simulink model "Robot2"  (R2019b)
settings: Solver=ode4  StartTime=0.0  StopTime=Tsim  FixedStep=Ts  RelTol=1e-3
values from neighbouring files (symbols this model uses):
  alfa = 20    [MAIN.m]
  delta = 0.1    [MAIN.m]
  gain = 1.0    (= 1)    [MAIN.m]
  Gname = ['G' num2str(grados) 'Rn']    [MAIN.m]
  IMname = ['InvMass' num2str(grados) 'Rn' ]    [MAIN.m]
  K = 0.1    [MAIN.m]
  lambda = 20    [MAIN.m]
  limD = -[60 40]'    [MAIN.m]
  limU = [60 40]'    [MAIN.m]
  Mname = ['Mass' num2str(grados) 'Rn' ]    [MAIN.m]
  P = 1    [MAIN.m]
  q0 = [0 0]'    [MAIN.m]
  q01 = q0+(Offset*pi/180)    [MAIN.m]
  qd0 = [0 0]'    [MAIN.m]
  Tg = 1e-3    (= 0.001)    [MAIN.m]
  Vname = ['V' num2str(grados) 'Rn' ]    [MAIN.m]
undefined symbols (not defined in the file or in its folder): smiData, X, Y, Z
libraries: sm_lib x16, nesl_utility x7
settings Model: Creator=AP34340  LastModifiedBy=AP34340
settings DataIOCC: SaveOutput=off  SignalLogging=off  DSMLogging=off  SaveTime=off  ReturnWorkspaceOutputs=off
settings OptimizationCC: LifeSpan=inf
settings DebuggingCC: SFExecutionAtInitializationDiag=none  ArithmeticOperatorsInVariantConditions=warning
settings HardwareCC: ProdBitPerSizeT=32  ProdBitPerPtrDiffT=32  ProdWordSize=32  ProdHWDeviceType=Specified
settings ModelReferenceCC: EnableParallelModelReferenceBuilds=on  ParallelModelReferenceMATLABWorkerInit=Load Top Model
settings SFSimCC: CustomCodeUndefinedFunction=UseInterfaceOnly
settings CodeAppCC: StateflowObjectComments=on
settings SimscapeCC: SimscapeNormalizeSystem=off

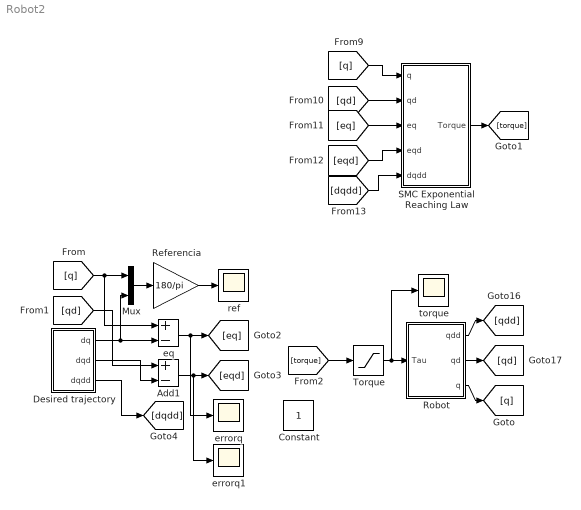
== system Robot2 ==
  Add1 : Sum  Inputs=+-
  Desired trajectory : Subsystem
  Mux : Mux  Inputs=2
  Referencia : Gain  Gain=180/pi
  Robot : Subsystem
  SMC Exponential Reaching Law : Subsystem
  Torque : Saturate  UpperLimit=limU  LowerLimit=limD
  eq : Sum  Inputs=+-
  errorq : Scope
  errorq1 : Scope
  ref : Scope
  torque : Scope
  Constant : Constant  IOType=siggen
  wires:
  [q] -> Mux/1, eq/1
  Desired trajectory/3(dqdd) -> [dqdd]
  [qd] -> Add1/1
  Desired trajectory/2(dqd) -> Add1/2
  Add1/1 -> errorq1/1, [eqd]
  Mux/1 -> Referencia/1
  Robot/1(qdd) -> [qdd]
  Torque/1 -> Robot/1(Tau), torque/1
  Referencia/1 -> ref/1
  eq/1 -> [eq], errorq/1
  Robot/2(qd) -> [qd]
  Robot/3(q) -> [q]
  Desired trajectory/1(dq) -> Mux/2, eq/2
  [torque] -> Torque/1
  [q] -> SMC Exponential Reaching Law/1(q)
  SMC Exponential Reaching Law/1(Torque) -> [torque]
  [qd] -> SMC Exponential Reaching Law/2(qd)
  [eqd] -> SMC Exponential Reaching Law/4(eqd)
  [dqdd] -> SMC Exponential Reaching Law/5(dqdd)
  [eq] -> SMC Exponential Reaching Law/3(eq)

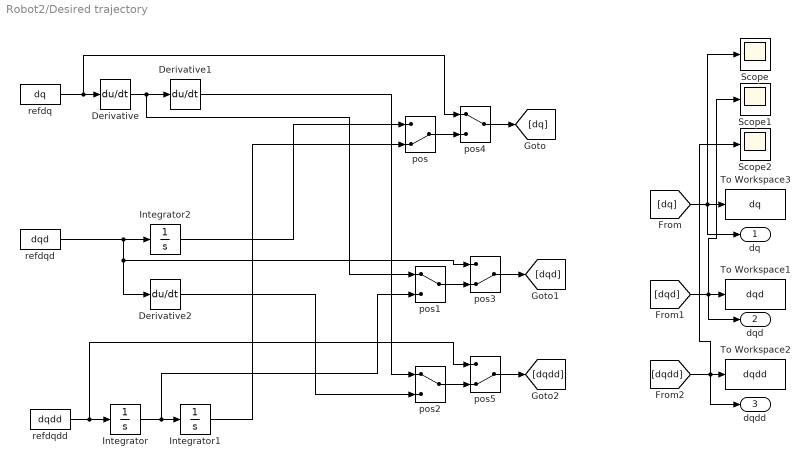
== system Robot2/Desired trajectory ==
  Derivative : Derivative
  Derivative1 : Derivative
  Derivative2 : Derivative
  Integrator : Integrator
  Integrator1 : Integrator  InitialCondition=q0
  Integrator2 : Integrator  InitialCondition=q0
  Scope : Scope
  Scope1 : Scope
  Scope2 : Scope
  To Workspace1 : ToWorkspace  VariableName=dqd  SampleTime=Tg
  To Workspace2 : ToWorkspace  VariableName=dqdd  SampleTime=Tg
  To Workspace3 : ToWorkspace  VariableName=dq  SampleTime=Tg
  pos : ManualSwitch  CurrentSetting=0
  pos1 : ManualSwitch
  pos2 : ManualSwitch
  pos3 : ManualSwitch  CurrentSetting=0
  pos4 : ManualSwitch
  pos5 : ManualSwitch  CurrentSetting=0
  refdq : FromWorkspace  VariableName=dq  SampleTime=0
  refdqd : FromWorkspace  VariableName=dqd  SampleTime=0
  refdqdd : FromWorkspace  VariableName=dqdd  SampleTime=0
  dq : Outport  VectorParamsAs1DForOutWhenUnconnected=off
  dqd : Outport  Port=2  VectorParamsAs1DForOutWhenUnconnected=off
  dqdd : Outport  Port=3  VectorParamsAs1DForOutWhenUnconnected=off
  wires:
  Integrator/1 -> pos1/2, Integrator1/1
  refdqdd/1 -> pos5/1, Integrator/1
  Derivative/1 -> pos1/1, Derivative1/1
  refdq/1 -> pos4/1, Derivative/1
  refdqd/1 -> Derivative2/1, pos3/1, Integrator2/1
  [dq] -> dq/1, Scope/1, To Workspace3/1
  [dqd] -> To Workspace1/1, Scope1/1, dqd/1
  [dqdd] -> Scope2/1, dqdd/1, To Workspace2/1
  pos4/1 -> [dq]
  pos3/1 -> [dqd]
  pos/1 -> pos4/2
  pos1/1 -> pos3/2
  pos2/1 -> pos5/2
  pos5/1 -> [dqdd]
  Integrator2/1 -> pos/1
  Integrator1/1 -> pos/2
  Derivative1/1 -> pos2/1
  Derivative2/1 -> pos2/2

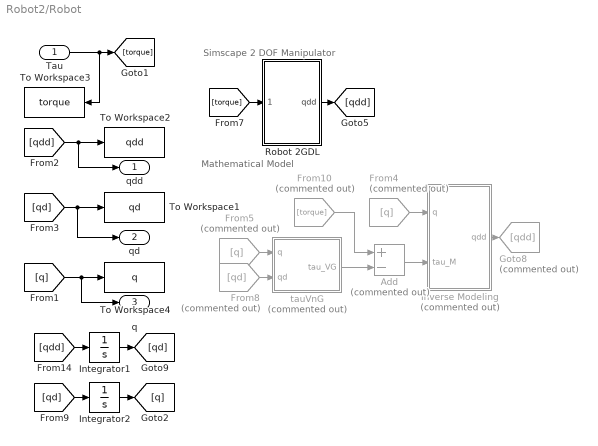
== system Robot2/Robot ==
  note: Mathematical Model
  note: Simscape 2 DOF Manipulator
  Tau : Inport
  " tauVnG" : Subsystem  Commented=on
  Add : Sum  Commented=on  Inputs=+-
  From10 : From  Commented=on  GotoTag=torque
  From4 : From  Commented=on  GotoTag=q
  From5 : From  Commented=on  GotoTag=q
  From8 : From  Commented=on  GotoTag=qd
  Goto8 : Goto  Commented=on  GotoTag=qdd
  Integrator1 : Integrator  InitialCondition=qd0
  Integrator2 : Integrator  InitialCondition=q01
  Inverse Modeling : Subsystem  Commented=on
  Robot 2GDL : Subsystem
  To Workspace1 : ToWorkspace  VariableName=qd  SampleTime=Tg
  To Workspace2 : ToWorkspace  VariableName=qdd  SampleTime=Tg
  To Workspace3 : ToWorkspace  VariableName=torque  SampleTime=Tg
  To Workspace4 : ToWorkspace  VariableName=q  SampleTime=Tg
  qdd : Outport  VectorParamsAs1DForOutWhenUnconnected=off
  qd : Outport  Port=2  VectorParamsAs1DForOutWhenUnconnected=off
  q : Outport  Port=3  VectorParamsAs1DForOutWhenUnconnected=off
  wires:
  [qdd] -> qdd/1, To Workspace2/1
  [qdd] -> Integrator1/1
  Integrator1/1 -> [qd]
  From4/1 -> Inverse Modeling/1(q)
  Add/1 -> Inverse Modeling/2(tau_M)
  Inverse Modeling/1(qdd) -> Goto8/1
  From5/1 -> " tauVnG"/1(q)
  " tauVnG"/1(tau_VG) -> Add/2
  From8/1 -> " tauVnG"/2(qd)
  Integrator2/1 -> [q]
  [qd] -> Integrator2/1
  From10/1 -> Add/1
  [q] -> q/1, To Workspace4/1
  Tau/1 -> [torque], To Workspace3/1
  [qd] -> qd/1, To Workspace1/1
  Robot 2GDL/1(qdd) -> [qdd]
  [torque] -> Robot 2GDL/1(torque)

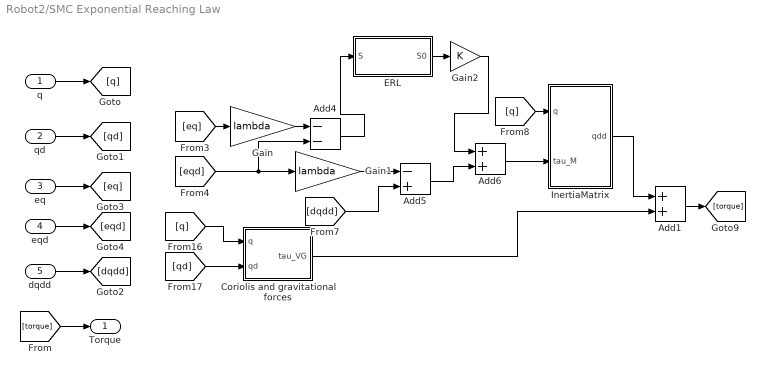
== system Robot2/SMC Exponential Reaching Law ==
  q : Inport
  qd : Inport  Port=2
  eq : Inport  Port=3
  eqd : Inport  Port=4
  dqdd : Inport  Port=5
  " Coriolis and gravitational forces" : Subsystem
  Add1 : Sum
  Add4 : Sum  Inputs=--
  Add5 : Sum  Inputs=-+
  Add6 : Sum
  ERL : Subsystem
  Gain : Gain  Gain=lambda
  Gain1 : Gain  Gain=lambda
  Gain2 : Gain  Gain=K
  InertiaMatrix : Subsystem
  Torque : Outport
  wires:
  [eqd] -> Gain1/1, Add4/2
  Gain1/1 -> Add5/1
  Gain/1 -> Add4/1
  Add5/1 -> Add6/2
  [dqdd] -> Add5/2
  [eq] -> Gain/1
  eqd/1 -> [eqd]
  eq/1 -> [eq]
  dqdd/1 -> [dqdd]
  [torque] -> Torque/1
  [q] -> " Coriolis and gravitational forces"/1(q)
  [qd] -> " Coriolis and gravitational forces"/2(qd)
  Add1/1 -> [torque]
  q/1 -> [q]
  qd/1 -> [qd]
  [q] -> InertiaMatrix/1(q)
  Gain2/1 -> Add6/1
  Add6/1 -> InertiaMatrix/2(tau_M)
  InertiaMatrix/1(qdd) -> Add1/1
  Add4/1 -> ERL/1(S)
  " Coriolis and gravitational forces"/1(tau_VG) -> Add1/2
  ERL/1(S0) -> Gain2/1

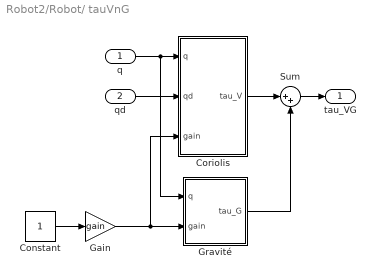
== system Robot2/Robot/ tauVnG ==
  q : Inport
  qd : Inport  Port=2
  Constant : Constant
  Coriolis : Subsystem
  Gain : Gain  Gain=gain
  Gravité : Subsystem
  Sum : Sum  Inputs=|++  SaturateOnIntegerOverflow=on  InputSameDT=on  OutDataTypeStr=Inherit: Same as first input
  tau_VG : Outport  VectorParamsAs1DForOutWhenUnconnected=off
  wires:
  q/1 -> Gravité/1(q), Coriolis/1(q)
  qd/1 -> Coriolis/2(qd)
  Coriolis/1(tau_V) -> Sum/1
  Gravité/1(tau_G) -> Sum/2
  Sum/1 -> tau_VG/1
  Gain/1 -> Gravité/2(gain), Coriolis/3(gain)
  Constant/1 -> Gain/1

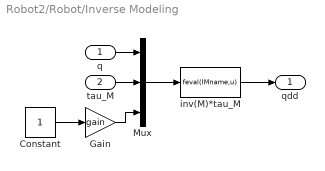
== system Robot2/Robot/Inverse Modeling ==
  q : Inport
  tau_M : Inport  Port=2
  Constant : Constant
  Gain : Gain  Gain=gain
  Mux : Mux  Inputs=3
  inv(M)*tau_M : MATLABFcn  MATLABFcn=feval(IMname,u)
  qdd : Outport  VectorParamsAs1DForOutWhenUnconnected=off
  wires:
  q/1 -> Mux/1
  tau_M/1 -> Mux/2
  Mux/1 -> inv(M)*tau_M/1
  inv(M)*tau_M/1 -> qdd/1
  Constant/1 -> Gain/1
  Gain/1 -> Mux/3

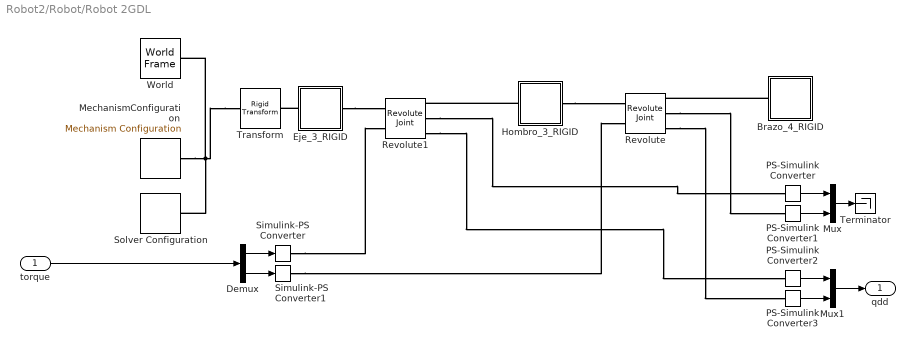
== system Robot2/Robot/Robot 2GDL ==
  torque : Inport
  Brazo_4_RIGID : Subsystem
  Demux : Demux  Outputs=2
  Eje_3_RIGID : Subsystem
  Hombro_3_RIGID : Subsystem
  MechanismConfiguration : sm_lib/Utilities/Mechanism Configuration  UniformGravity=Constant  GravityVector=[0 0 -9.80665]  GravityUnits=m/s^2  LinearizationDelta=0.001
  Mux : Mux  Inputs=2
  Mux1 : Mux  Inputs=2
  PS-Simulink Converter{,1..3} (4 alike) : nesl_utility/PS-Simulink Converter  PhysicalDomain=network_engine_domain  SubClassName=ps_output  LeftPortType=input  RightPortType=output  PseudoPeriodic=off  Frequencies=[]  Unit=1  AffineConversion=off
  Revolute : sm_lib/Joints/Revolute Joint  JointMode=Normal  SenseConstraintForce=off  SenseConstraintForceX=off  SenseConstraintForceY=off  SenseConstraintForceZ=off  SenseConstraintTorque=off  SenseConstraintTorqueX=off  SenseConstraintTorqueY=off  SenseConstraintTorqueZ=off  SenseTotalForce=off  SenseTotalForceX=off  SenseTotalForceY=off  SenseTotalForceZ=off  SenseTotalTorque=off  SenseTotalTorqueX=off  SenseTotalTorqueY=off  SenseTotalTorqueZ=off  CompositeWrenchDir=FollowerOnBase  CompositeWrenchFrame=BaseFrame  EquilibriumPosition=0  EquilibriumPositionUnits=rad  SpringStiffness=0  SpringStiffnessUnits=N*m/rad  DampingCoefficient=0  DampingCoefficientUnits=N*m/(rad/s)  TorqueActuationMode=InputTorque  MotionActuationMode=ComputedMotion  SensePosition=on  SenseVelocity=off  SenseAcceleration=on  SenseTorqueForce=off  SenseLowerLimitTorqueForce=off  SenseUpperLimitTorqueForce=off  LowerLimitSpecify=off  LowerLimitBound=-90  LowerLimitBoundUnits=deg  LowerLimitStiffness=1e4  LowerLimitStiffnessUnits=N*m/deg  LowerLimitDamping=10  LowerLimitDampingUnits=N*m/(deg/s)  LowerLimitTransitionRegionWidth=0.1  LowerLimitTransitionRegionWidthUnits=deg  UpperLimitSpecify=off  UpperLimitBound=90  UpperLimitBoundUnits=deg  UpperLimitStiffness=1e4  UpperLimitStiffnessUnits=N*m/deg  UpperLimitDamping=10  UpperLimitDampingUnits=N*m/(deg/s)  UpperLimitTransitionRegionWidth=0.1  UpperLimitTransitionRegionWidthUnits=deg  PositionTargetSpecify=on  PositionTargetPriority=Low  PositionTargetValue=smiData.RevoluteJoint(2).Rz.Pos  PositionTargetValueUnits=deg  VelocityTargetSpecify=on  VelocityTargetPriority=Low  VelocityTargetValue=smiData.RevoluteJoint(2).Rz.Vel  VelocityTargetValueUnits=deg/s
  Revolute1 : sm_lib/Joints/Revolute Joint  JointMode=Normal  SenseConstraintForce=off  SenseConstraintForceX=off  SenseConstraintForceY=off  SenseConstraintForceZ=off  SenseConstraintTorque=off  SenseConstraintTorqueX=off  SenseConstraintTorqueY=off  SenseConstraintTorqueZ=off  SenseTotalForce=off  SenseTotalForceX=off  SenseTotalForceY=off  SenseTotalForceZ=off  SenseTotalTorque=off  SenseTotalTorqueX=off  SenseTotalTorqueY=off  SenseTotalTorqueZ=off  CompositeWrenchDir=FollowerOnBase  CompositeWrenchFrame=BaseFrame  EquilibriumPosition=0  EquilibriumPositionUnits=rad  SpringStiffness=0  SpringStiffnessUnits=N*m/rad  DampingCoefficient=0  DampingCoefficientUnits=N*m/(rad/s)  TorqueActuationMode=InputTorque  MotionActuationMode=ComputedMotion  SensePosition=on  SenseVelocity=off  SenseAcceleration=on  SenseTorqueForce=off  SenseLowerLimitTorqueForce=off  SenseUpperLimitTorqueForce=off  LowerLimitSpecify=off  LowerLimitBound=-90  LowerLimitBoundUnits=deg  LowerLimitStiffness=1e4  LowerLimitStiffnessUnits=N*m/deg  LowerLimitDamping=10  LowerLimitDampingUnits=N*m/(deg/s)  LowerLimitTransitionRegionWidth=0.1  LowerLimitTransitionRegionWidthUnits=deg  UpperLimitSpecify=off  UpperLimitBound=90  UpperLimitBoundUnits=deg  UpperLimitStiffness=1e4  UpperLimitStiffnessUnits=N*m/deg  UpperLimitDamping=10  UpperLimitDampingUnits=N*m/(deg/s)  UpperLimitTransitionRegionWidth=0.1  UpperLimitTransitionRegionWidthUnits=deg  PositionTargetSpecify=on  PositionTargetPriority=Low  PositionTargetValue=smiData.RevoluteJoint(1).Rz.Pos  PositionTargetValueUnits=deg  VelocityTargetSpecify=on  VelocityTargetPriority=Low  VelocityTargetValue=smiData.RevoluteJoint(1).Rz.Vel  VelocityTargetValueUnits=deg/s
  Simulink-PS Converter : nesl_utility/Simulink-PS Converter  PhysicalDomain=network_engine_domain  SubClassName=ps_input  LeftPortType=input  RightPortType=output  PseudoPeriodic=off  Frequencies=[]  NoiseDistribution=none  NoiseParameters=[]  Unit=1  AffineConversion=off  FilteringAndDerivatives=provide  SimscapeFilterOrder=1  InputFilterTimeConstant=0.001  UdotUserProvided=0
  Simulink-PS Converter1 : nesl_utility/Simulink-PS Converter  PhysicalDomain=network_engine_domain  SubClassName=ps_input  LeftPortType=input  RightPortType=output  PseudoPeriodic=off  Frequencies=[]  NoiseDistribution=none  NoiseParameters=[]  Unit=1  AffineConversion=off  FilteringAndDerivatives=provide  SimscapeFilterOrder=1  InputFilterTimeConstant=0.001  UdotUserProvided=0
  Solver Configuration : nesl_utility/Solver Configuration  PhysicalDomain=network_engine_domain  SubClassName=solver  LeftPortType=input  RightPortType=generic  Tones=[]  Harmonics=[]  SimulateNoise=off  Profile=off  UseLocalSampling=off  EnableSwitchedLinearOptims=on  FrequencyDomain=off  UseCCode=off  RelTol=0.001  AbsTol=1e-06  MinStep=1e-09  ToWorkspace=off  RevertToSquareIcSolve=off  NumHomotopyIterations=100  PhasorMode=off  PhasorModeNumHarmonics=1  DoDC=off  ResidualTolerance=1e-09  UseLocalSolver=off  LocalSolverChoice=NE_BACKWARD_EULER_ADVANCER  LocalSolverSampleTime=0.001  DoFixedCost=off  MaxNonlinIter=3  MaxModeIter=2  LinearAlgebra=auto  EquationFormulation=NE_TIME_EF  DelaysMemoryBudget=1024  AutomaticFiltering=on  FilteringTimeConstant=0.001  PartitionStorageMethod=AS_NEEDED  PartitionMemoryBudget=1024  PartitionMethod=FAST
  Terminator : Terminator
  Transform : sm_lib/Frames and Transforms/Rigid Transform  TranslationMethod=Cartesian  TranslationStandardOffset=0  TranslationLengthUnit=mm  TranslationStandardAxis=+Z  TranslationCartesianOffset=smiData.RigidTransform(5).translation  TranslationROffset=0  TranslationROffsetUnits=m  TranslationZOffset=0  TranslationZOffsetUnits=m  TranslationThetaOffset=0  TranslationThetaOffsetUnits=deg  RotationMethod=ArbitraryAxis  RotationAngleUnits=rad  RotationStandardAxis=+Z  RotationAngle=smiData.RigidTransform(5).angle  RotationArbitraryAxis=smiData.RigidTransform(5).axis  FollAlignAxisA=+X  BaseAlignAxisA=+Y  FollAlignAxisB=+Y  BaseAlignAxisB=+Z  RotationSequenceAxes=FollowerAxes  RotationSequence=XYX  RotationSequenceAngles=[0 0 0]  RotationSequenceAnglesUnits=deg  RotationMatrix=[1 0 0; 0 1 0; 0 0 1]
  World : sm_lib/Frames and Transforms/World Frame
  qdd : Outport  VectorParamsAs1DForOutWhenUnconnected=off
  wires:
  Demux/1 -> Simulink-PS Converter/1
  Demux/2 -> Simulink-PS Converter1/1
  PS-Simulink Converter/1 -> Mux/1
  PS-Simulink Converter1/1 -> Mux/2
  torque/1 -> Demux/1
  PS-Simulink Converter3/1 -> Mux1/2
  PS-Simulink Converter2/1 -> Mux1/1
  Mux1/1 -> qdd/1
  Mux/1 -> Terminator/1
  connections:
  Brazo_4_RIGID/LConn1 -- Revolute/RConn1
  Transform/LConn1 -- MechanismConfiguration/RConn1 -- Solver Configuration/RConn1 -- World/RConn1
  Eje_3_RIGID/LConn1 -- Transform/RConn1
  Eje_3_RIGID/RConn1 -- Revolute1/LConn1
  Hombro_3_RIGID/LConn1 -- Revolute1/RConn1
  Hombro_3_RIGID/RConn1 -- Revolute/LConn1
  Simulink-PS Converter/RConn1 -- Revolute1/LConn2
  Simulink-PS Converter1/RConn1 -- Revolute/LConn2
  Revolute1/RConn2 -- PS-Simulink Converter/LConn1
  Revolute/RConn2 -- PS-Simulink Converter1/LConn1
  Revolute1/RConn3 -- PS-Simulink Converter2/LConn1
  Revolute/RConn3 -- PS-Simulink Converter3/LConn1

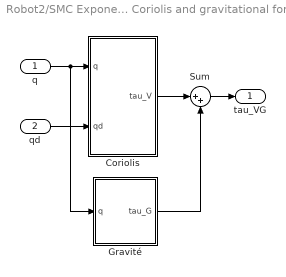
== system Robot2/SMC Exponential Reaching Law/ Coriolis and gravitational forces ==
  q : Inport
  qd : Inport  Port=2
  Coriolis : Subsystem
  Gravité : Subsystem
  Sum : Sum  Inputs=|++  SaturateOnIntegerOverflow=on  InputSameDT=on  OutDataTypeStr=Inherit: Same as first input
  tau_VG : Outport  VectorParamsAs1DForOutWhenUnconnected=off
  wires:
  q/1 -> Gravité/1(q), Coriolis/1(q)
  qd/1 -> Coriolis/2(qd)
  Coriolis/1(tau_V) -> Sum/1
  Gravité/1(tau_G) -> Sum/2
  Sum/1 -> tau_VG/1

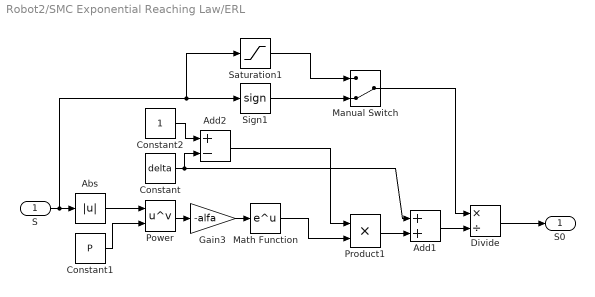
== system Robot2/SMC Exponential Reaching Law/ERL ==
  S : Inport
  Abs : Abs
  Add1 : Sum
  Add2 : Sum  Inputs=+-
  Constant : Constant  Value=delta
  Constant1 : Constant  Value=P
  Constant2 : Constant
  Divide : Product  Inputs=*/
  Gain3 : Gain  Gain=-alfa
  Manual Switch : ManualSwitch  CurrentSetting=0
  Math Function : Math  SignedPower=off  SaturateOnIntegerOverflow=on
  Power : Math  Operator=pow  SignedPower=off  SaturateOnIntegerOverflow=on
  Product1 : Product
  Saturation1 : Saturate  UpperLimit=1  LowerLimit=-1
  Sign1 : Signum
  S0 : Outport
  wires:
  Product1/1 -> Add1/2
  Add2/1 -> Product1/1
  Math Function/1 -> Product1/2
  Constant/1 -> Add1/1, Add2/2
  Constant2/1 -> Add2/1
  Constant1/1 -> Power/2
  Abs/1 -> Power/1
  S/1 -> Saturation1/1, Sign1/1, Abs/1
  Add1/1 -> Divide/2
  Divide/1 -> S0/1
  Power/1 -> Gain3/1
  Gain3/1 -> Math Function/1
  Sign1/1 -> Manual Switch/2
  Saturation1/1 -> Manual Switch/1
  Manual Switch/1 -> Divide/1

== system Robot2/SMC Exponential Reaching Law/InertiaMatrix ==
  q : Inport
  tau_M : Inport  Port=2
  M*tau : MATLABFcn  MATLABFcn=feval(Mname,u)
  Mux : Mux  Inputs=2
  qdd : Outport  VectorParamsAs1DForOutWhenUnconnected=off
  wires:
  q/1 -> Mux/1
  Mux/1 -> M*tau/1
  tau_M/1 -> Mux/2
  M*tau/1 -> qdd/1

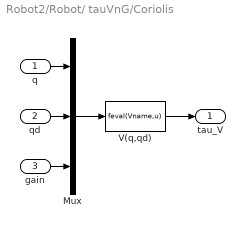
== system Robot2/Robot/ tauVnG/Coriolis ==
  q : Inport
  qd : Inport  Port=2
  gain : Inport  Port=3
  Mux : Mux  Inputs=3
  V(q,qd) : MATLABFcn  MATLABFcn=feval(Vname,u)
  tau_V : Outport  VectorParamsAs1DForOutWhenUnconnected=off
  wires:
  q/1 -> Mux/1
  qd/1 -> Mux/2
  V(q,qd)/1 -> tau_V/1
  Mux/1 -> V(q,qd)/1
  gain/1 -> Mux/3

== system Robot2/Robot/ tauVnG/Gravité ==
  q : Inport
  gain : Inport  Port=2
  G(q) : MATLABFcn  MATLABFcn=feval(Gname,u)
  Mux : Mux  Inputs=2
  tau_G : Outport  VectorParamsAs1DForOutWhenUnconnected=off
  wires:
  G(q)/1 -> tau_G/1
  q/1 -> Mux/1
  gain/1 -> Mux/2
  Mux/1 -> G(q)/1

== system Robot2/Robot/Robot 2GDL/Brazo_4_RIGID ==
  ReferenceFrame : sm_lib/Frames and Transforms/Reference Frame
  Solid : sm_lib/Body Elements/File Solid  ExtGeomFileName=Brazo_Predeterminado_sldprt.STEP  UnitType=FromFile  ExtGeomFileUnits=m  StepReaderType=HEX  ExportEntireGeometry=off  InertiaType=Custom  Mass=smiData.Solid(2).mass  MassUnits=kg  CenterOfMass=smiData.Solid(2).CoM  CenterOfMassUnits=m  MomentsOfInertia=smiData.Solid(2).MoI  MomentsOfInertiaUnits=kg*m^2  ProductsOfInertia=smiData.Solid(2).PoI  ProductsOfInertiaUnits=kg*m^2  BasedOnType=Density  Density=1000  DensityUnits=kg/m^3  DoExposeReferenceFrame=on  SerializedFrames=<Frames/>  GraphicType=FromGeometry  MarkerShape=Sphere  MarkerSize=10  GraphicVisPropType=SimpleVisualProperties  GraphicDiffuseColor=smiData.Solid(2).color  GraphicSpecularColor=[0.5 0.5 0.5 1.0]  GraphicAmbientColor=[0.15 0.15 0.15 1.0]  GraphicEmissiveColor=[0.0 0.0 0.0 1.0]  GraphicShininess=75  GraphicOpacity=smiData.Solid(2).opacity
  Transform : sm_lib/Frames and Transforms/Rigid Transform  TranslationMethod=Cartesian  TranslationStandardOffset=0  TranslationLengthUnit=mm  TranslationStandardAxis=+Z  TranslationCartesianOffset=smiData.RigidTransform(2).translation  TranslationROffset=0  TranslationROffsetUnits=m  TranslationZOffset=0  TranslationZOffsetUnits=m  TranslationThetaOffset=0  TranslationThetaOffsetUnits=deg  RotationMethod=ArbitraryAxis  RotationAngleUnits=rad  RotationStandardAxis=+Z  RotationAngle=smiData.RigidTransform(2).angle  RotationArbitraryAxis=smiData.RigidTransform(2).axis  FollAlignAxisA=+X  BaseAlignAxisA=+Y  FollAlignAxisB=+Y  BaseAlignAxisB=+Z  RotationSequenceAxes=FollowerAxes  RotationSequence=XYX  RotationSequenceAngles=[0 0 0]  RotationSequenceAnglesUnits=deg  RotationMatrix=[1 0 0; 0 1 0; 0 0 1]
  F : PMIOPort  Side=Left
  connections:
  Solid/RConn1 -- ReferenceFrame/RConn1 -- Transform/LConn1
  Transform/RConn1 -- F/RConn1

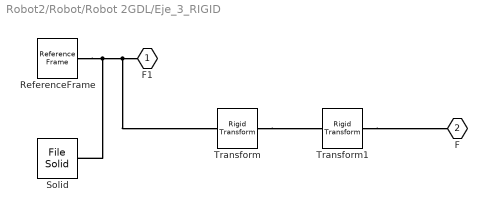
== system Robot2/Robot/Robot 2GDL/Eje_3_RIGID ==
  ReferenceFrame : sm_lib/Frames and Transforms/Reference Frame
  Solid : sm_lib/Body Elements/File Solid  ExtGeomFileName=Eje_Predeterminado_sldprt.STEP  UnitType=FromFile  ExtGeomFileUnits=m  StepReaderType=HEX  ExportEntireGeometry=off  InertiaType=Custom  Mass=smiData.Solid(1).mass  MassUnits=kg  CenterOfMass=smiData.Solid(1).CoM  CenterOfMassUnits=in  MomentsOfInertia=smiData.Solid(1).MoI  MomentsOfInertiaUnits=kg*in^2  ProductsOfInertia=smiData.Solid(1).PoI  ProductsOfInertiaUnits=kg*in^2  BasedOnType=Density  Density=1000  DensityUnits=kg/m^3  DoExposeReferenceFrame=on  SerializedFrames=<Frames/>  GraphicType=FromGeometry  MarkerShape=Sphere  MarkerSize=10  GraphicVisPropType=SimpleVisualProperties  GraphicDiffuseColor=smiData.Solid(1).color  GraphicSpecularColor=[0.5 0.5 0.5 1.0]  GraphicAmbientColor=[0.15 0.15 0.15 1.0]  GraphicEmissiveColor=[0.0 0.0 0.0 1.0]  GraphicShininess=75  GraphicOpacity=smiData.Solid(1).opacity
  Transform : sm_lib/Frames and Transforms/Rigid Transform  TranslationMethod=Cartesian  TranslationStandardOffset=0  TranslationLengthUnit=mm  TranslationStandardAxis=+Z  TranslationCartesianOffset=smiData.RigidTransform(3).translation  TranslationROffset=0  TranslationROffsetUnits=m  TranslationZOffset=0  TranslationZOffsetUnits=m  TranslationThetaOffset=0  TranslationThetaOffsetUnits=deg  RotationMethod=ArbitraryAxis  RotationAngleUnits=rad  RotationStandardAxis=+Z  RotationAngle=smiData.RigidTransform(3).angle  RotationArbitraryAxis=smiData.RigidTransform(3).axis  FollAlignAxisA=+X  BaseAlignAxisA=+Y  FollAlignAxisB=+Y  BaseAlignAxisB=+Z  RotationSequenceAxes=FollowerAxes  RotationSequence=XYX  RotationSequenceAngles=[0 0 0]  RotationSequenceAnglesUnits=deg  RotationMatrix=[1 0 0; 0 1 0; 0 0 1]
  Transform1 : sm_lib/Frames and Transforms/Rigid Transform  TranslationMethod=Cartesian  TranslationStandardOffset=0  TranslationLengthUnit=mm  TranslationStandardAxis=+Z  TranslationCartesianOffset=[0 0 0]  TranslationROffset=0  TranslationROffsetUnits=m  TranslationZOffset=0  TranslationZOffsetUnits=m  TranslationThetaOffset=0  TranslationThetaOffsetUnits=deg  RotationMethod=ArbitraryAxis  RotationAngleUnits=rad  RotationStandardAxis=+Z  RotationAngle=pi/2  RotationArbitraryAxis=[0 0 -1]  FollAlignAxisA=+X  BaseAlignAxisA=+Y  FollAlignAxisB=+Y  BaseAlignAxisB=+Z  RotationSequenceAxes=FollowerAxes  RotationSequence=XYX  RotationSequenceAngles=[0 0 0]  RotationSequenceAnglesUnits=deg  RotationMatrix=[1 0 0; 0 1 0; 0 0 1]
  F1 : PMIOPort  Side=Left
  F : PMIOPort  Port=2  Side=Right
  connections:
  Solid/RConn1 -- ReferenceFrame/RConn1 -- Transform/LConn1 -- F1/RConn1
  Transform1/RConn1 -- F/RConn1
  Transform/RConn1 -- Transform1/LConn1

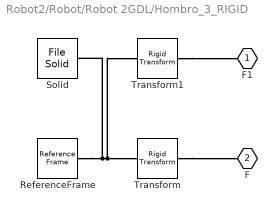
== system Robot2/Robot/Robot 2GDL/Hombro_3_RIGID ==
  ReferenceFrame : sm_lib/Frames and Transforms/Reference Frame
  Solid : sm_lib/Body Elements/File Solid  ExtGeomFileName=Hombro_Predeterminado_sldprt.STEP  UnitType=FromFile  ExtGeomFileUnits=m  StepReaderType=HEX  ExportEntireGeometry=off  InertiaType=Custom  Mass=smiData.Solid(3).mass  MassUnits=kg  CenterOfMass=smiData.Solid(3).CoM  CenterOfMassUnits=m  MomentsOfInertia=smiData.Solid(3).MoI  MomentsOfInertiaUnits=kg*m^2  ProductsOfInertia=smiData.Solid(3).PoI  ProductsOfInertiaUnits=kg*m^2  BasedOnType=Density  Density=1000  DensityUnits=kg/m^3  DoExposeReferenceFrame=on  SerializedFrames=<Frames/>  GraphicType=FromGeometry  MarkerShape=Sphere  MarkerSize=10  GraphicVisPropType=SimpleVisualProperties  GraphicDiffuseColor=smiData.Solid(3).color  GraphicSpecularColor=[0.5 0.5 0.5 1.0]  GraphicAmbientColor=[0.15 0.15 0.15 1.0]  GraphicEmissiveColor=[0.0 0.0 0.0 1.0]  GraphicShininess=75  GraphicOpacity=smiData.Solid(3).opacity
  Transform : sm_lib/Frames and Transforms/Rigid Transform  TranslationMethod=Cartesian  TranslationStandardOffset=0  TranslationLengthUnit=mm  TranslationStandardAxis=+Z  TranslationCartesianOffset=smiData.RigidTransform(1).translation  TranslationROffset=0  TranslationROffsetUnits=m  TranslationZOffset=0  TranslationZOffsetUnits=m  TranslationThetaOffset=0  TranslationThetaOffsetUnits=deg  RotationMethod=ArbitraryAxis  RotationAngleUnits=rad  RotationStandardAxis=+Z  RotationAngle=smiData.RigidTransform(1).angle  RotationArbitraryAxis=smiData.RigidTransform(1).axis  FollAlignAxisA=+X  BaseAlignAxisA=+Y  FollAlignAxisB=+Y  BaseAlignAxisB=+Z  RotationSequenceAxes=FollowerAxes  RotationSequence=XYX  RotationSequenceAngles=[0 0 0]  RotationSequenceAnglesUnits=deg  RotationMatrix=[1 0 0; 0 1 0; 0 0 1]
  Transform1 : sm_lib/Frames and Transforms/Rigid Transform  TranslationMethod=Cartesian  TranslationStandardOffset=0  TranslationLengthUnit=mm  TranslationStandardAxis=+Z  TranslationCartesianOffset=smiData.RigidTransform(4).translation  TranslationROffset=0  TranslationROffsetUnits=m  TranslationZOffset=0  TranslationZOffsetUnits=m  TranslationThetaOffset=0  TranslationThetaOffsetUnits=deg  RotationMethod=ArbitraryAxis  RotationAngleUnits=rad  RotationStandardAxis=+Z  RotationAngle=smiData.RigidTransform(4).angle  RotationArbitraryAxis=smiData.RigidTransform(4).axis  FollAlignAxisA=+X  BaseAlignAxisA=+Y  FollAlignAxisB=+Y  BaseAlignAxisB=+Z  RotationSequenceAxes=FollowerAxes  RotationSequence=XYX  RotationSequenceAngles=[0 0 0]  RotationSequenceAnglesUnits=deg  RotationMatrix=[1 0 0; 0 1 0; 0 0 1]
  F1 : PMIOPort  Side=Left
  F : PMIOPort  Port=2  Side=Right
  connections:
  Solid/RConn1 -- ReferenceFrame/RConn1 -- Transform/LConn1 -- Transform1/LConn1
  Transform/RConn1 -- F/RConn1
  Transform1/RConn1 -- F1/RConn1

== system Robot2/SMC Exponential Reaching Law/ Coriolis and gravitational forces/Coriolis ==
  q : Inport
  qd : Inport  Port=2
  Mux : Mux  Inputs=2
  V(q,qd) : MATLABFcn  MATLABFcn=feval(Vname,u)  OutputDimensions=grados
  tau_V : Outport  VectorParamsAs1DForOutWhenUnconnected=off
  wires:
  q/1 -> Mux/1
  qd/1 -> Mux/2
  V(q,qd)/1 -> tau_V/1
  Mux/1 -> V(q,qd)/1

== system Robot2/SMC Exponential Reaching Law/ Coriolis and gravitational forces/Gravité ==
  q : Inport
  G(q) : MATLABFcn  MATLABFcn=feval(Gname,u)  OutputDimensions=grados
  tau_G : Outport  VectorParamsAs1DForOutWhenUnconnected=off
  wires:
  G(q)/1 -> tau_G/1
  q/1 -> G(q)/1
